simulink model "sinwave"  (R2023b)
settings: Solver=VariableStepAuto  StartTime=0.0  StopTime=20  RelTol=1e-3
libraries: simulink x1
settings Model: Creator=yasinsensoy  LastModifiedBy=yasinsensoy

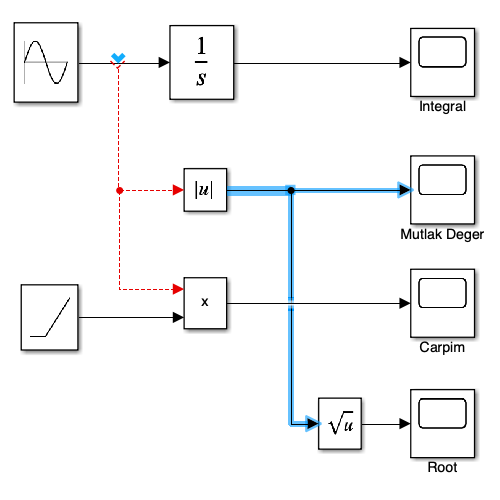
[thumbnail: Simulink's stored preview of the top-level diagram]
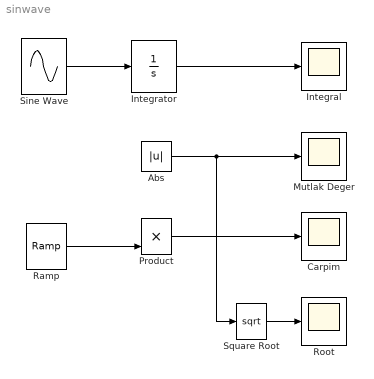
== system sinwave ==
  Abs : Abs  SaturateOnIntegerOverflow=off
  Carpim : Scope
  Integral : Scope
  Integrator : Integrator
  Mutlak Deger : Scope
  Product : Product
  Ramp : simulink/Sources/Ramp  slope=1  start=0  InitialOutput=0
  Root : Scope
  Sine Wave : Sin  SampleTime=0
  Square Root : Sqrt
  wires:
  Sine Wave/1 -> Integrator/1
  Integrator/1 -> Integral/1
  ? -> Product/1, Abs/1
  Abs/1 -> Square Root/1, Mutlak Deger/1
  Ramp/1 -> Product/2
  Product/1 -> Carpim/1
  Square Root/1 -> Root/1
